simulink model "DemuxTwoOutput"  (R2024b)
settings: Solver=VariableStepAuto  StartTime=0.0  StopTime=10.0  RelTol=1e-3
settings Model: Creator=ferbe  LastModifiedBy=ferbe

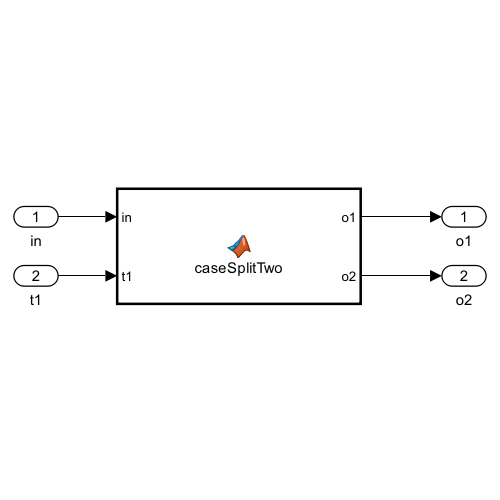
[thumbnail: Simulink's stored preview of the top-level diagram]
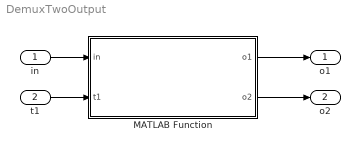
== system DemuxTwoOutput ==
  in : Inport
  t1 : Inport  Port=2
  MATLAB Function : MATLAB Function  TreatAsAtomicUnit=on
  o1 : Outport
  o2 : Outport  Port=2
  wires:
  in/1 -> MATLAB Function/1(in)
  t1/1 -> MATLAB Function/2(t1)
  MATLAB Function/1(o1) -> o1/1
  MATLAB Function/2(o2) -> o2/1

== matlab function DemuxTwoOutput/MATLAB Function ==
  data: in input; o1 output; t1 input; o2 output
function [o1, o2] = caseSplitTwo(in, t1)

    o1 = -1;
    o2 = -1;
    x =100 * rand;
    if 0  <= x && x < t1
    
        o1 = in;
    
    else
    
        o2 = in;
    
    end
end
